simulink model "SF5_5_2_jc0751"  (R2016b)
settings: Solver=VariableStepAuto  StartTime=0.0  StopTime=10.0  RelTol=1e-3  EnableMultiTasking=on
settings Model: Creator=amyyang  LastModifiedBy=amyyang
settings DataIOCC: LimitDataPoints=on
settings OptimizationCC: LifeSpan=inf
settings DebuggingCC: AllowSymbolicDim=off  SFUnexpectedBacktrackingDiag=warning  SFNoUnconditionalDefaultTransitionDiag=warning  SFExecutionAtInitializationDiag=none
settings ModelReferenceCC: PropagateSignalLabelsOutOfModel=off
settings GRTTargetCC: TargetLangStandard=C89/C90 (ANSI)
settings ConfigComp: CovMetricSettings=dw  CovHtmlReporting=on  CovSaveCumulativeToWorkspaceVar=on  CovSaveSingleToWorkspaceVar=on  CovExternalEMLEnable=off

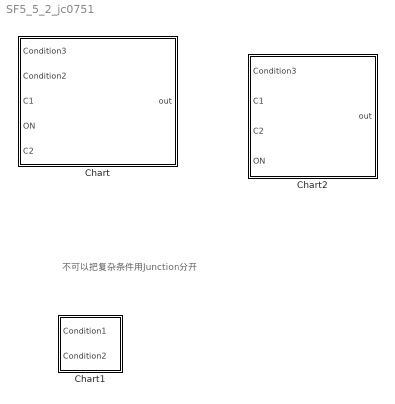
== system SF5_5_2_jc0751 ==
  note: 不可以把复杂条件用Junction分开
  Chart : Stateflow chart  TreatAsAtomicUnit=on
  Chart1 : Stateflow chart  TreatAsAtomicUnit=on
  Chart2 : Stateflow chart  TreatAsAtomicUnit=on

== stateflow chart SF5_5_2_jc0751/Chart1 ==
  state A [parallel]
    settings: executionOrder=1
    state Correct
    state C
    (default) -> Correct
    Correct -> C : [ Condition1 && Condition2]
  state B [parallel]
    settings: executionOrder=2
    note: 不可以把复杂条件用Junction分开
    state InCorrect1
    state C2
    (default) -> InCorrect1
    InCorrect1 -> (junction 238) : [ Condition1 ]
    (junction 238) -> C2 : [ Condition2 ]
  data: Condition1 input; Condition2 input

== stateflow chart SF5_5_2_jc0751/Chart2 ==
  state A1 [parallel]
    settings: executionOrder=8
    state Correct1
    state Correct2
    state Correct3
    (default) -> Correct1
    Correct1 -> Correct2 [order 2]
    Correct1 -> (junction 288) [order 1]
    (junction 288) -> (junction 289) [order 1] : [ (C1 == ON) && ( C2 == ON)]
    (junction 288) -> Correct3 [order 2] : [ Condition2]
        | {
        |  out = 1;
        | }
    (junction 289) -> Correct3 : {
        |  out = 2;
        | }
  note: Diagnostics诊断配置 Stateflow可以配置检查 Unexpected backtracking
  state B1 [parallel]
    settings: executionOrder=10
    note: 不允许，否则当 CI==ON，而C2 == OFF，就会产生
        | Backtracking
    state InCorrect9
    state Correct7
    state Correct8
    (default) -> InCorrect9
    InCorrect9 -> Correct7 [order 2] : [Condition3]
    InCorrect9 -> (junction 290) [order 1]
    (junction 290) -> (junction 291) [order 1] : [ (C1 == ON) ]
    (junction 291) -> (junction 292) : [ ( C2 == ON)]
    (junction 290) -> Correct8 [order 2] : [ Condition2]
        | {
        |  out = 1;
        | }
    (junction 292) -> Correct8 : {
        |  out = 3;
        | }
  state C1 [parallel]
    settings: executionOrder=9
    state Correct4
    state Correct5
    note: 所有的Junction都有分支
    state Correct6
    (default) -> Correct4
    Correct4 -> Correct5 [order 2] : [Condition3]
    Correct4 -> (junction 293) [order 1]
    (junction 293) -> (junction 294) [order 1] : [ (C1 == ON) ]
    (junction 294) -> (junction 295) [order 1] : [ ( C2 == ON)]
    (junction 293) -> Correct6 [order 2] : [ Condition2]
        | {
        |  out = 1;
        | }
    (junction 294) -> Correct6 [order 2] : {
        |  out = 2;
        | }
    (junction 295) -> Correct6 : {
        |  out = 3;
        | }
  note: Diagnostics诊断配置 Stateflow可以配置检查 Unexpected backtracking
  state A [parallel]
    settings: executionOrder=1
    state Correct12
    state Correct13
    state Correct14
    (default) -> Correct12
    Correct12 -> Correct13 [order 2] : [Condition3]
    Correct12 -> Correct14 [order 1] : [ (C1 == ON) && ( C2 == ON)]
        | {
        |  out = 2;
        | }
  state B [parallel]
    settings: executionOrder=2
    state Correct9
    state Correct10
    note: 跟左边是等效的
    state Correct11
    (default) -> Correct9
    Correct9 -> Correct10 [order 2] : [Condition3]
    Correct9 -> (junction 151) [order 1]
    (junction 151) -> (junction 154) : [ (C1 == ON) && ( C2 == ON)]
    (junction 154) -> Correct11 : {
        |  out = 2;
        | }
  state E [parallel]
    settings: executionOrder=3
    state InCorrect21
    state Correct23
    note: 这样就会产生回流
    state Correct22
    (default) -> InCorrect21
    InCorrect21 -> Correct23 [order 2] : [Condition3]
    InCorrect21 -> (junction 194) [order 1]
    (junction 194) -> (junction 205) : [ (C1 == ON) ]
    (junction 205) -> (junction 197) : [ ( C2 == ON)]
    (junction 197) -> Correct22 : {
        |  out = 3;
        | }
  state C [parallel]
    settings: executionOrder=4
    state Correct18
    state Correct19
    state Correct20
    (default) -> Correct18
    Correct18 -> Correct19 [order 2] : [Condition3]
    Correct18 -> (junction 182) [order 1] : [ (C1 == ON) ]
    (junction 182) -> (junction 189) [order 1] : [ ( C2 == ON)]
    (junction 182) -> Correct20 [order 2] : {
        |  out = 2;
        | }
    (junction 189) -> Correct20 : {
        |  out = 3;
        | }
  state D [parallel]
    settings: executionOrder=5
    state Correct16
    state Correct15
    note: 跟左边是等效的
    state Correct17
    (default) -> Correct16
    Correct16 -> Correct15 [order 2] : [Condition3]
    Correct16 -> (junction 167) [order 1]
    (junction 167) -> (junction 171) : [ (C1 == ON) ]
    (junction 171) -> (junction 178) [order 1] : [ ( C2 == ON)]
    (junction 171) -> Correct17 [order 2] : {
        |  out = 2;
        | }
    (junction 178) -> Correct17 : {
        |  out = 3;
        | }
  state F [parallel]
    settings: executionOrder=6
    state Correct27
    state Correct26
    (default) -> Correct27
    Correct27 -> (junction 226) [order 1]
    Correct27 -> (junction 227) [order 2] : [Condition3 && ( C2 == ON)]
    (junction 226) -> (junction 227) : [ (C1 == ON) && ( C2 == ON) ]
    (junction 227) -> Correct26 : {
        |  out = 3;
        | }
  state G [parallel]
    settings: executionOrder=7
    state InCorrect24
    note: 比如这种形式，就要改成左边
    state Correct25
    (default) -> InCorrect24
    InCorrect24 -> (junction 209) [order 1]
    InCorrect24 -> (junction 217) [order 2] : [Condition3]
    (junction 209) -> (junction 217) : [ (C1 == ON) ]
    (junction 217) -> (junction 214) : [ ( C2 == ON)]
    (junction 214) -> Correct25 : {
        |  out = 3;
        | }
  data: Condition3 input; out output; C1 input; C2 input; ON input

== stateflow chart SF5_5_2_jc0751/Chart ==
  data: Condition3 input; Condition2 input; out output; C1 input; ON input; C2 input
